simulink model "Integrated_Model"  (R2019a)
settings: Solver=FixedStepAuto  StartTime=0.0  StopTime=1000  FixedStep=0.1  RelTol=1e-3
settings Model: Creator=Kore  LastModifiedBy=User

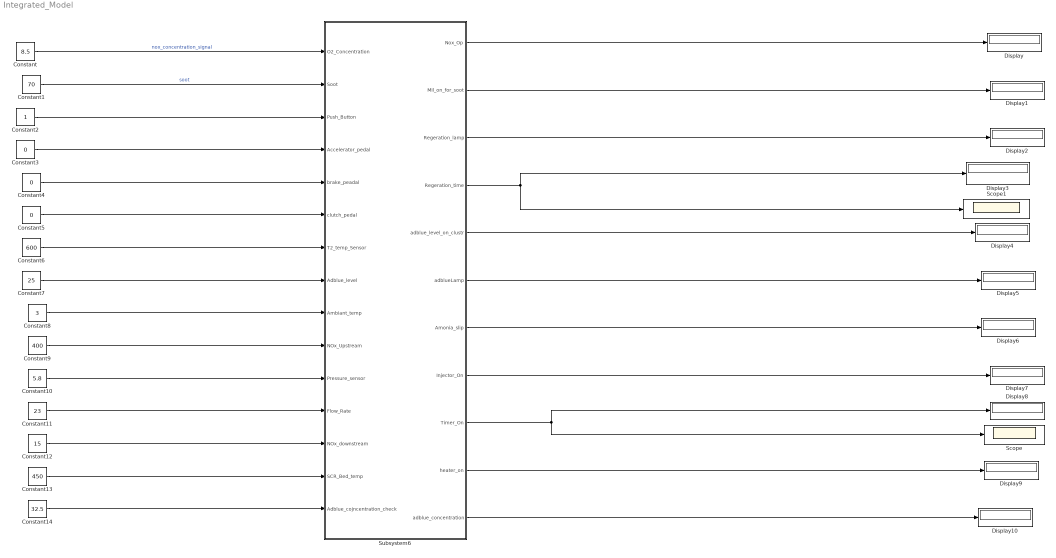
== system Integrated_Model ==
  Constant : Constant  Value=8.5
  Constant1 : Constant  Value=70
  Constant10 : Constant  Value=5.8
  Constant11 : Constant  Value=23
  Constant12 : Constant  Value=15
  Constant13 : Constant  Value=450
  Constant14 : Constant  Value=32.5
  Constant2 : Constant
  Constant3 : Constant  Value=0
  Constant4 : Constant  Value=0
  Constant5 : Constant  Value=0
  Constant6 : Constant  Value=600
  Constant7 : Constant  Value=25
  Constant8 : Constant  Value=3
  Constant9 : Constant  Value=400
  Display{,1..10} (11 alike) : Display
  Scope : Scope
  Scope1 : Scope
  Subsystem6 : Subsystem
  wires:
  Constant/1 -> Subsystem6/1(O2_Concentration)  "nox_concentration_signal"
  Constant1/1 -> Subsystem6/2(Soot)  "soot"
  Constant2/1 -> Subsystem6/3(Push_Button)
  Constant3/1 -> Subsystem6/4(Accelerator_pedal)
  Constant4/1 -> Subsystem6/5(brake_peadal)
  Constant5/1 -> Subsystem6/6(clutch_pedal)
  Constant6/1 -> Subsystem6/7(T2_temp_Sensor)
  Constant7/1 -> Subsystem6/8(Adblue_level)
  Constant8/1 -> Subsystem6/9(Ambiant_temp)
  Constant9/1 -> Subsystem6/10(NOx_Upstream)
  Constant10/1 -> Subsystem6/11(Pressure_sensor)
  Constant11/1 -> Subsystem6/12(Flow_Rate)
  Constant12/1 -> Subsystem6/13(NOx_downstream)
  Constant13/1 -> Subsystem6/14(SCR_Bed_temp)
  Subsystem6/1(Nox_Op) -> Display/1
  Subsystem6/2(MIl_on_for_soot) -> Display1/1
  Subsystem6/3(Regeration_lamp) -> Display2/1
  Subsystem6/4(Regeration_time) -> Scope1/1, Display3/1
  Subsystem6/5(adblue_level_on_clustr) -> Display4/1
  Subsystem6/7(Amonia_slip) -> Display6/1
  Subsystem6/8(Injector_On) -> Display7/1
  Subsystem6/9(Timer_On) -> Display8/1, Scope/1
  Subsystem6/10(heater_on) -> Display9/1
  Subsystem6/11(adblue_concentration) -> Display10/1
  Constant14/1 -> Subsystem6/15(Adblue_cojncentration_check)
  Subsystem6/6(adblueLamp) -> Display5/1

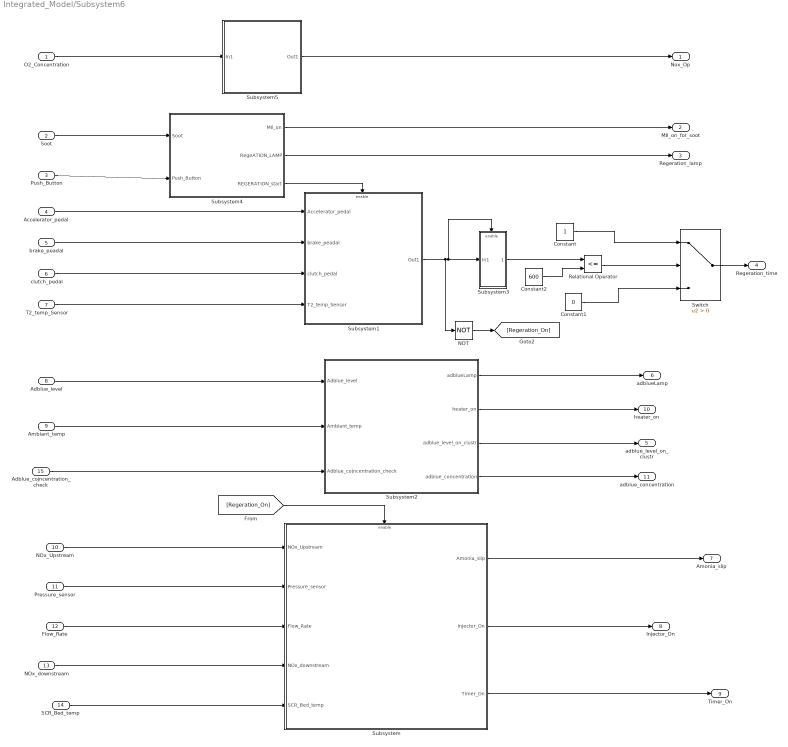
== system Integrated_Model/Subsystem6 ==
  O2_Concentration : Inport
  Soot : Inport  Port=2
  Push_Button : Inport  Port=3
  Accelerator_pedal : Inport  Port=4
  brake_peadal : Inport  Port=5
  clutch_pedal : Inport  Port=6
  T2_temp_Sensor : Inport  Port=7
  Adblue_level : Inport  Port=8
  Ambiant_temp : Inport  Port=9
  NOx_Upstream : Inport  Port=10
  Pressure_sensor : Inport  Port=11
  Flow_Rate : Inport  Port=12
  NOx_downstream : Inport  Port=13
  SCR_Bed_temp : Inport  Port=14
  Adblue_cojncentration_check : Inport  Port=15
  Constant : Constant
  Constant1 : Constant  Value=0
  Constant2 : Constant  Value=600
  NOT : Logic  Operator=NOT  IconShape=distinctive  AllPortsSameDT=off  OutDataTypeStr=boolean
  Relational Operator : RelationalOperator  Operator=<=  OutDataTypeStr=boolean  RndMeth=Simplest
  Subsystem : Subsystem
  Subsystem1 : Subsystem
  Subsystem2 : Subsystem
  Subsystem3 : Subsystem
  Subsystem4 : Subsystem
  Subsystem5 : Subsystem
  Switch : Switch  Criteria=u2 > Threshold
  Nox_Op : Outport
  MIl_on_for_soot : Outport  Port=2
  Regeration_lamp : Outport  Port=3
  Regeration_time : Outport  Port=4
  adblue_level_on_clustr : Outport  Port=5
  adblueLamp : Outport  Port=6
  Amonia_slip : Outport  Port=7
  Injector_On : Outport  Port=8
  Timer_On : Outport  Port=9
  heater_on : Outport  Port=10
  adblue_concentration : Outport  Port=11
  wires:
  T2_temp_Sensor/1 -> Subsystem1/4(T2_temp_Sensor)
  NOT/1 -> [Regeration_On]
  Subsystem/3(Timer_On) -> Timer_On/1
  Subsystem1/1(Out1) -> Subsystem3/Enable, Subsystem3/1(In1), NOT/1
  Push_Button/1 -> Subsystem4/2(Push_Button)
  Subsystem4/3(REGERATION_start) -> Subsystem1/Enable
  Switch/1 -> Regeration_time/1
  Subsystem/1(Amonia_slip) -> Amonia_slip/1
  NOx_Upstream/1 -> Subsystem/1(NOx_Upstream)
  Subsystem3/1(Out1) -> Relational Operator/1
  Subsystem5/1(Out1) -> Nox_Op/1
  Subsystem4/2(RegeATION_LAMP) -> Regeration_lamp/1
  [Regeration_On] -> Subsystem/Enable
  Adblue_level/1 -> Subsystem2/1(Adblue_level)
  O2_Concentration/1 -> Subsystem5/1(In1)
  clutch_pedal/1 -> Subsystem1/3(clutch_pedal)
  Accelerator_pedal/1 -> Subsystem1/1(Accelerator_pedal)
  Flow_Rate/1 -> Subsystem/3(Flow_Rate)
  Soot/1 -> Subsystem4/1(Soot)
  Pressure_sensor/1 -> Subsystem/2(Pressure_sensor)
  Subsystem/2(Injector_On) -> Injector_On/1
  NOx_downstream/1 -> Subsystem/4(NOx_downstream)
  SCR_Bed_temp/1 -> Subsystem/5(SCR_Bed_temp)
  Subsystem4/1(MIl_on) -> MIl_on_for_soot/1
  brake_peadal/1 -> Subsystem1/2("brake_peadal ")
  Ambiant_temp/1 -> Subsystem2/2(Ambiant_temp)
  Subsystem2/1(adblueLamp) -> adblueLamp/1
  Subsystem2/3(adblue_level_on_clustr) -> adblue_level_on_clustr/1
  Subsystem2/2(heater_on) -> heater_on/1
  Relational Operator/1 -> Switch/2
  Constant/1 -> Switch/1
  Constant1/1 -> Switch/3
  Constant2/1 -> Relational Operator/2
  Adblue_cojncentration_check/1 -> Subsystem2/3(Adblue_cojncentration_check)
  Subsystem2/4(adblue_concentration) -> adblue_concentration/1

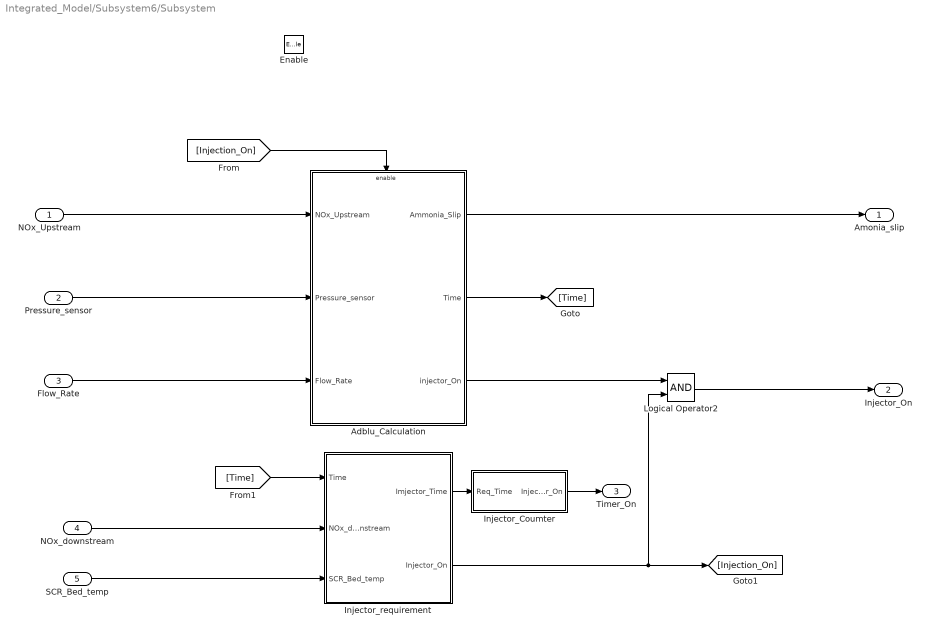
== system Integrated_Model/Subsystem6/Subsystem ==
  NOx_Upstream : Inport
  Pressure_sensor : Inport  Port=2
  Flow_Rate : Inport  Port=3
  NOx_downstream : Inport  Port=4
  SCR_Bed_temp : Inport  Port=5
  Enable : EnablePort
  Adblu_Calculation : Subsystem
  Injector_Coumter : Subsystem
  Injector_requirement : Subsystem
  Logical Operator2 : Logic  AllPortsSameDT=off  OutDataTypeStr=boolean
  Amonia_slip : Outport
  Injector_On : Outport  Port=2
  Timer_On : Outport  Port=3
  wires:
  Adblu_Calculation/2(Time) -> [Time]
  [Time] -> Injector_requirement/1(Time)
  Injector_Coumter/1(Injector_On) -> Timer_On/1
  Logical Operator2/1 -> Injector_On/1
  Injector_requirement/2(Injector_On) -> Logical Operator2/2, [Injection_On]
  Injector_requirement/1(Imjector_Time) -> Injector_Coumter/1(Req_Time)
  Adblu_Calculation/3(injector_On) -> Logical Operator2/1
  [Injection_On] -> Adblu_Calculation/Enable
  Adblu_Calculation/1(Ammonia_Slip) -> Amonia_slip/1
  NOx_downstream/1 -> Injector_requirement/2(NOx_downstream)
  NOx_Upstream/1 -> Adblu_Calculation/1(NOx_Upstream)
  SCR_Bed_temp/1 -> Injector_requirement/3(SCR_Bed_temp)
  Pressure_sensor/1 -> Adblu_Calculation/2(Pressure_sensor)
  Flow_Rate/1 -> Adblu_Calculation/3(Flow_Rate)

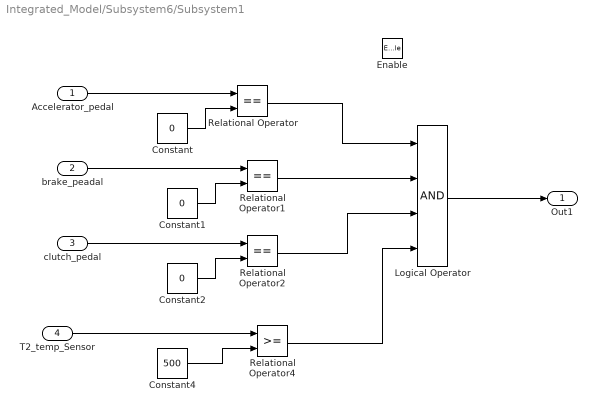
== system Integrated_Model/Subsystem6/Subsystem1 ==
  Accelerator_pedal : Inport
  "brake_peadal " : Inport  Port=2
  clutch_pedal : Inport  Port=3
  T2_temp_Sensor : Inport  Port=4
  Enable : EnablePort  StatesWhenEnabling=reset
  Constant : Constant  Value=0
  Constant1 : Constant  Value=0
  Constant2 : Constant  Value=0
  Constant4 : Constant  Value=500
  Logical Operator : Logic  Inputs=4  AllPortsSameDT=off  OutDataTypeStr=boolean
  Relational Operator : RelationalOperator  Operator===  OutDataTypeStr=boolean  RndMeth=Simplest
  Relational Operator1 : RelationalOperator  Operator===  OutDataTypeStr=boolean  RndMeth=Simplest
  Relational Operator2 : RelationalOperator  Operator===  OutDataTypeStr=boolean  RndMeth=Simplest
  Relational Operator4 : RelationalOperator  OutDataTypeStr=boolean  RndMeth=Simplest
  Out1 : Outport
  wires:
  Constant/1 -> Relational Operator/2
  Accelerator_pedal/1 -> Relational Operator/1
  "brake_peadal "/1 -> Relational Operator1/1
  Constant1/1 -> Relational Operator1/2
  Constant2/1 -> Relational Operator2/2
  clutch_pedal/1 -> Relational Operator2/1
  Relational Operator/1 -> Logical Operator/1
  Relational Operator1/1 -> Logical Operator/2
  Relational Operator2/1 -> Logical Operator/3
  T2_temp_Sensor/1 -> Relational Operator4/1
  Constant4/1 -> Relational Operator4/2
  Logical Operator/1 -> Out1/1
  Relational Operator4/1 -> Logical Operator/4

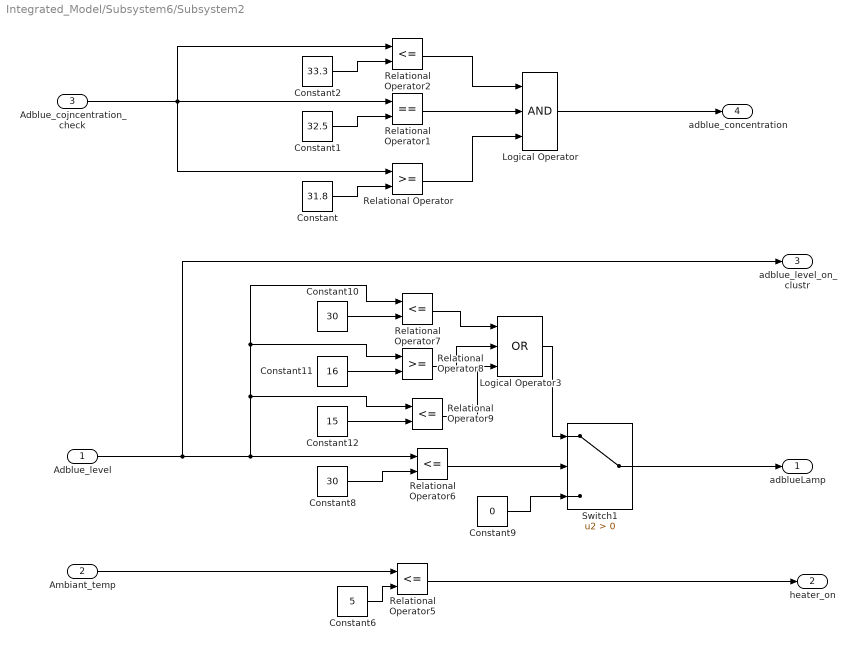
== system Integrated_Model/Subsystem6/Subsystem2 ==
  Adblue_level : Inport
  Ambiant_temp : Inport  Port=2
  Adblue_cojncentration_check : Inport  Port=3
  Constant : Constant  Value=31.8
  Constant1 : Constant  Value=32.5
  Constant10 : Constant  Value=30
  Constant11 : Constant  Value=16
  Constant12 : Constant  Value=15
  Constant2 : Constant  Value=33.3
  Constant6 : Constant  Value=5  OutDataTypeStr=int8
  Constant8 : Constant  Value=30
  Constant9 : Constant  Value=0
  Logical Operator : Logic  Inputs=3  AllPortsSameDT=off  OutDataTypeStr=boolean
  Logical Operator3 : Logic  Operator=OR  Inputs=3  AllPortsSameDT=off  OutDataTypeStr=boolean
  Relational Operator : RelationalOperator  OutDataTypeStr=boolean  RndMeth=Simplest
  Relational Operator1 : RelationalOperator  Operator===  OutDataTypeStr=boolean  RndMeth=Simplest
  Relational Operator{2,5..7,9} (5 alike) : RelationalOperator  Operator=<=  OutDataTypeStr=boolean  RndMeth=Simplest
  Relational Operator8 : RelationalOperator  OutDataTypeStr=boolean  RndMeth=Simplest
  Switch1 : Switch  Criteria=u2 > Threshold
  adblueLamp : Outport
  heater_on : Outport  Port=2
  adblue_level_on_clustr : Outport  Port=3
  adblue_concentration : Outport  Port=4
  wires:
  Logical Operator3/1 -> Switch1/1
  Constant9/1 -> Switch1/3
  Adblue_level/1 -> adblue_level_on_clustr/1, Relational Operator6/1, Relational Operator9/1, Relational Operator8/1, Relational Operator7/1
  Constant10/1 -> Relational Operator7/2
  Constant11/1 -> Relational Operator8/2
  Constant8/1 -> Relational Operator6/2
  Relational Operator8/1 -> Logical Operator3/2
  Constant12/1 -> Relational Operator9/2
  Relational Operator9/1 -> Logical Operator3/3
  Relational Operator6/1 -> Switch1/2
  Relational Operator7/1 -> Logical Operator3/1
  Constant6/1 -> Relational Operator5/2
  Relational Operator5/1 -> heater_on/1
  Switch1/1 -> adblueLamp/1
  Ambiant_temp/1 -> Relational Operator5/1
  Constant/1 -> Relational Operator/2
  Constant1/1 -> Relational Operator1/2
  Adblue_cojncentration_check/1 -> Relational Operator/1, Relational Operator2/1, Relational Operator1/1
  Constant2/1 -> Relational Operator2/2
  Relational Operator2/1 -> Logical Operator/1
  Relational Operator1/1 -> Logical Operator/2
  Relational Operator/1 -> Logical Operator/3
  Logical Operator/1 -> adblue_concentration/1

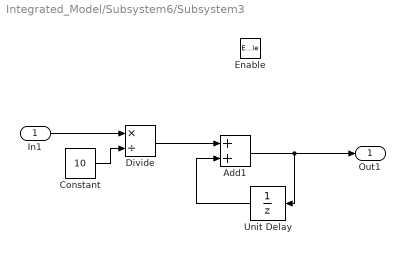
== system Integrated_Model/Subsystem6/Subsystem3 ==
  In1 : Inport
  Enable : EnablePort  StatesWhenEnabling=reset
  Add1 : Sum  OutDataTypeStr=double  RndMeth=Round
  Constant : Constant  Value=10
  Divide : Product  Inputs=*/
  Unit Delay : UnitDelay  InitialCondition=0.1  SampleTime=-1  HasFrameUpgradeWarning=on
  Out1 : Outport
  wires:
  Add1/1 -> Out1/1, Unit Delay/1
  Unit Delay/1 -> Add1/2
  In1/1 -> Divide/1
  Divide/1 -> Add1/1
  Constant/1 -> Divide/2

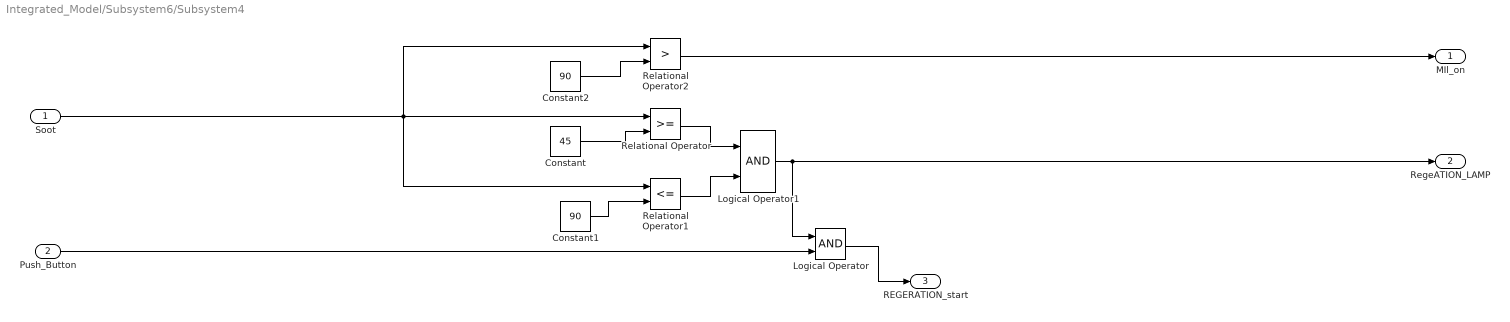
== system Integrated_Model/Subsystem6/Subsystem4 ==
  Soot : Inport
  Push_Button : Inport  Port=2
  Constant : Constant  Value=45
  Constant1 : Constant  Value=90
  Constant2 : Constant  Value=90
  Logical Operator : Logic  AllPortsSameDT=off  OutDataTypeStr=boolean
  Logical Operator1 : Logic  AllPortsSameDT=off  OutDataTypeStr=boolean
  Relational Operator : RelationalOperator  OutDataTypeStr=boolean  RndMeth=Simplest
  Relational Operator1 : RelationalOperator  Operator=<=  OutDataTypeStr=boolean  RndMeth=Simplest
  Relational Operator2 : RelationalOperator  Operator=>  OutDataTypeStr=boolean  RndMeth=Simplest
  MIl_on : Outport
  RegeATION_LAMP : Outport  Port=2
  REGERATION_start : Outport  Port=3
  wires:
  Soot/1 -> Relational Operator1/1, Relational Operator2/1, Relational Operator/1
  Logical Operator/1 -> REGERATION_start/1
  Logical Operator1/1 -> RegeATION_LAMP/1, Logical Operator/1
  Constant2/1 -> Relational Operator2/2
  Push_Button/1 -> Logical Operator/2
  Constant1/1 -> Relational Operator1/2
  Constant/1 -> Relational Operator/2
  Relational Operator1/1 -> Logical Operator1/2
  Relational Operator2/1 -> MIl_on/1
  Relational Operator/1 -> Logical Operator1/1

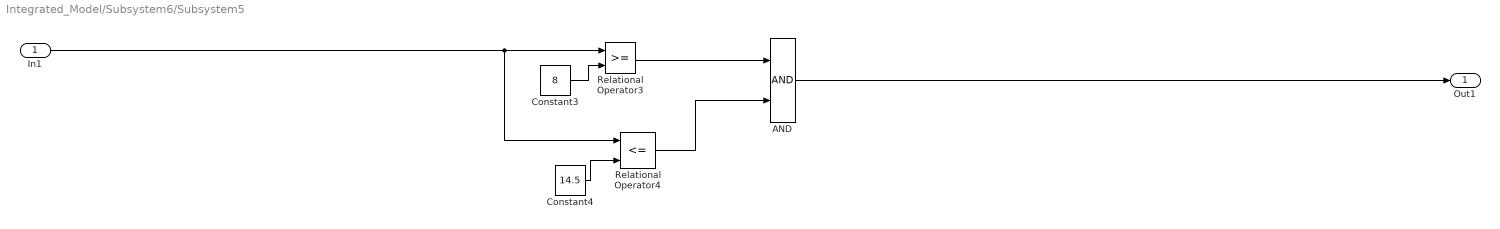
== system Integrated_Model/Subsystem6/Subsystem5 ==
  In1 : Inport
  AND : Logic  AllPortsSameDT=off  OutDataTypeStr=boolean
  Constant3 : Constant  Value=8
  Constant4 : Constant  Value=14.5
  Relational Operator3 : RelationalOperator  OutDataTypeStr=boolean  RndMeth=Simplest
  Relational Operator4 : RelationalOperator  Operator=<=  OutDataTypeStr=boolean  RndMeth=Simplest
  Out1 : Outport
  wires:
  Constant3/1 -> Relational Operator3/2
  Relational Operator3/1 -> AND/1
  AND/1 -> Out1/1
  In1/1 -> Relational Operator4/1, Relational Operator3/1
  Constant4/1 -> Relational Operator4/2
  Relational Operator4/1 -> AND/2

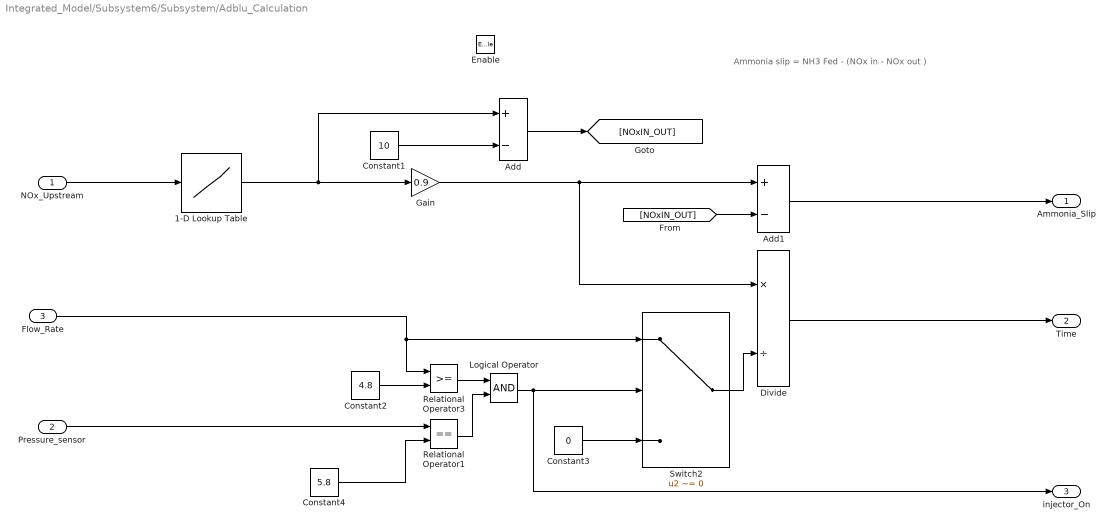
== system Integrated_Model/Subsystem6/Subsystem/Adblu_Calculation ==
  note: Ammonia slip = NH3 Fed - (NOx in - NOx out )
  NOx_Upstream : Inport
  Pressure_sensor : Inport  Port=2
  Flow_Rate : Inport  Port=3
  Enable : EnablePort  StatesWhenEnabling=reset
  1-D Lookup Table : Lookup_n-D  NumberOfTableDimensions=1  BreakpointsForDimension1=|  BreakpointsForDimension1DataTypeStr=double  Table=|  TableDataTypeStr=double  IntermediateResultsDataTypeStr=double  InternalRulePriority=Speed  OutDataTypeStr=double  RndMeth=Simplest  FractionDataTypeStr=double  InputSameDT=on
      BreakpointsForDimension1=|
      | [10
      | 70
      | 77.6
      | 80.4
      | 86.4
      | 99.6
      | 108
      | 117.6
      | 127.2
      | 136.8
      | 149.3
      | 158.3
      | 163.3
      | 168.3
      | 175.3
      | 181.5
      | 187.7
      | 193.9
      | 200.1
      | 206.3
      | 212.85
      | 223.5
      | 233.15
      | 242.8
      | 255.45
      | 264.9
      | 275.35
      | 285.8
      | 296.25
      | 306.7
      | 317.15
      | 327.6
      | 338.05
      | 348.5
      | 358.95
      | 369.4
      | 379.85
      | 390.3
      | 400.75
      | 411.2
      | 421.65
      | 432.1
      | 442.55
      | 453
      | 463.45
      | 473.9
      | 484.35
      | 494.8
      | 505.25
      | 515.7
      | 526.15
      | 536.6
      | 547.05
      | 557.5
      | 567.95
      | 578.4
      | 588.85
      | 599.3
      | 609.75
      | 620.2
      | 630.65
      | 641.1
      | 651.55
      | 662
      | 672.45
      | 682.9
      | 693.35
      | 703.8
      | ]
      Table=|
      | [10
      | 70
      | 77.6
      | 80.4
      | 86.4
      | 99.6
      | 108
      | 117.6
      | 127.2
      | 136.8
      | 149.3
      | 158.3
      | 163.3
      | 168.3
      | 175.3
      | 181.5
      | 187.7
      | 193.9
      | 200.1
      | 206.3
      | 212.85
      | 223.5
      | 233.15
      | 242.8
      | 255.45
      | 264.9
      | 275.35
      | 285.8
      | 296.25
      | 306.7
      | 317.15
      | 327.6
      | 338.05
      | 348.5
      | 358.95
      | 369.4
      | 379.85
      | 390.3
      | 400.75
      | 411.2
      | 421.65
      | 432.1
      | 442.55
      | 453
      | 463.45
      | 473.9
      | 484.35
      | 494.8
      | 505.25
      | 515.7
      | 526.15
      | 536.6
      | 547.05
      | 557.5
      | 567.95
      | 578.4
      | 588.85
      | 599.3
      | 609.75
      | 620.2
      | 630.65
      | 641.1
      | 651.55
      | 662
      | 672.45
      | 682.9
      | 693.35
      | 703.8
      | ]
  Add : Sum  Inputs=+-
  Add1 : Sum  Inputs=+-
  Constant1 : Constant  Value=10
  Constant2 : Constant  Value=4.8
  Constant3 : Constant  Value=0
  Constant4 : Constant  Value=5.8
  Divide : Product  Inputs=*/  OutDataTypeStr=double  RndMeth=Round
  Gain : Gain  Gain=0.9
  Logical Operator : Logic  AllPortsSameDT=off  OutDataTypeStr=boolean
  Relational Operator1 : RelationalOperator  Operator===  OutDataTypeStr=boolean  RndMeth=Simplest
  Relational Operator3 : RelationalOperator  OutDataTypeStr=boolean  RndMeth=Simplest
  Switch2 : Switch  Criteria=u2 ~= 0
  Ammonia_Slip : Outport
  Time : Outport  Port=2
  injector_On : Outport  Port=3
  wires:
  Pressure_sensor/1 -> Relational Operator1/1
  Add/1 -> [NOxIN_OUT]
  Constant1/1 -> Add/2
  Relational Operator1/1 -> Logical Operator/2
  Constant4/1 -> Relational Operator1/2
  NOx_Upstream/1 -> 1-D Lookup Table/1
  Constant2/1 -> Relational Operator3/2
  Relational Operator3/1 -> Logical Operator/1
  Constant3/1 -> Switch2/3
  Switch2/1 -> Divide/2
  Logical Operator/1 -> injector_On/1, Switch2/2
  [NOxIN_OUT] -> Add1/2
  Flow_Rate/1 -> Relational Operator3/1, Switch2/1
  Add1/1 -> Ammonia_Slip/1
  Gain/1 -> Divide/1, Add1/1
  Divide/1 -> Time/1
  1-D Lookup Table/1 -> Gain/1, Add/1

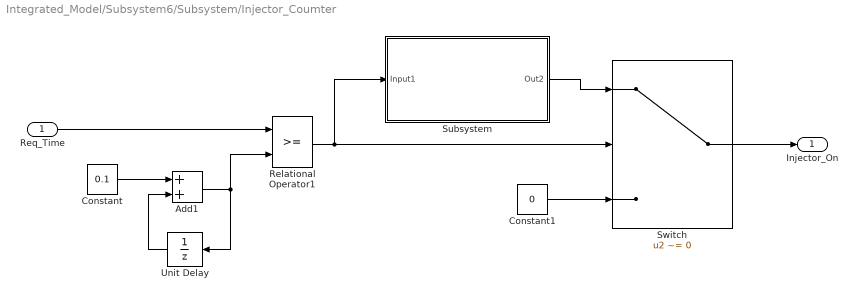
== system Integrated_Model/Subsystem6/Subsystem/Injector_Coumter ==
  Req_Time : Inport
  Add1 : Sum
  Constant : Constant  Value=0.1
  Constant1 : Constant  Value=0
  Relational Operator1 : RelationalOperator  OutDataTypeStr=boolean  RndMeth=Simplest
  Subsystem : Subsystem
  Switch : Switch  Criteria=u2 ~= 0
  Unit Delay : UnitDelay  SampleTime=-1  HasFrameUpgradeWarning=on
  Injector_On : Outport
  wires:
  Constant1/1 -> Switch/3
  Unit Delay/1 -> Add1/2
  Constant/1 -> Add1/1
  Add1/1 -> Unit Delay/1, Relational Operator1/2
  Subsystem/1(Out2) -> Switch/1
  Req_Time/1 -> Relational Operator1/1
  Switch/1 -> Injector_On/1
  Relational Operator1/1 -> Subsystem/1(Input1), Switch/2

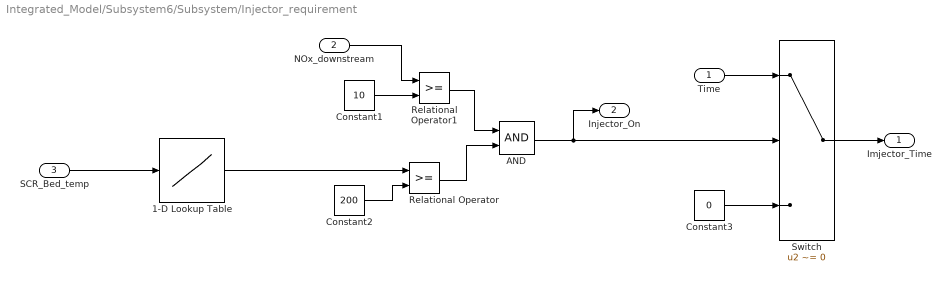
== system Integrated_Model/Subsystem6/Subsystem/Injector_requirement ==
  Time : Inport
  NOx_downstream : Inport  Port=2
  SCR_Bed_temp : Inport  Port=3
  1-D Lookup Table : Lookup_n-D  NumberOfTableDimensions=1  BreakpointsForDimension1=[1:10:650]  BreakpointsForDimension2=[1:1:500]  BreakpointsForDimension1DataTypeStr=double  Table=[1:10:650]  TableDataTypeStr=double  IntermediateResultsDataTypeStr=double  InternalRulePriority=Speed  OutDataTypeStr=double  RndMeth=Simplest  FractionDataTypeStr=double  InputSameDT=on
  AND : Logic  AllPortsSameDT=off  OutDataTypeStr=boolean
  Constant1 : Constant  Value=10
  Constant2 : Constant  Value=200
  Constant3 : Constant  Value=0
  Relational Operator : RelationalOperator  OutDataTypeStr=boolean  RndMeth=Simplest
  Relational Operator1 : RelationalOperator  OutDataTypeStr=boolean  RndMeth=Simplest
  Switch : Switch  Criteria=u2 ~= 0
  Imjector_Time : Outport
  Injector_On : Outport  Port=2
  wires:
  Constant1/1 -> Relational Operator1/2
  Constant2/1 -> Relational Operator/2
  Constant3/1 -> Switch/3
  1-D Lookup Table/1 -> Relational Operator/1
  AND/1 -> Injector_On/1, Switch/2
  Time/1 -> Switch/1
  Relational Operator1/1 -> AND/1
  Relational Operator/1 -> AND/2
  SCR_Bed_temp/1 -> 1-D Lookup Table/1
  Switch/1 -> Imjector_Time/1
  NOx_downstream/1 -> Relational Operator1/1

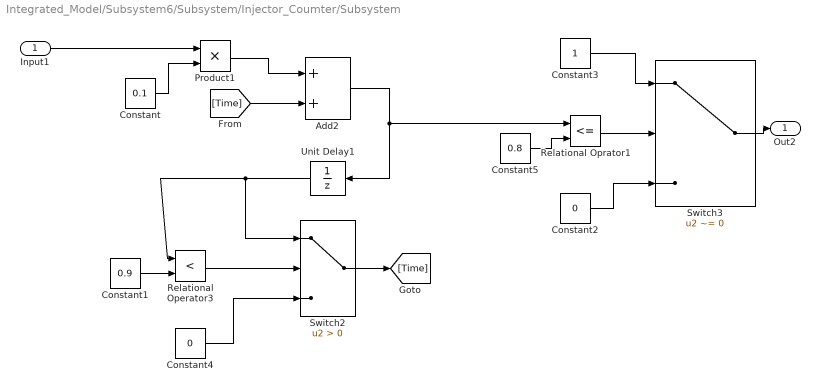
== system Integrated_Model/Subsystem6/Subsystem/Injector_Coumter/Subsystem ==
  Input1 : Inport
  Add2 : Sum
  Constant : Constant  Value=0.1
  Constant1 : Constant  Value=0.9
  Constant2 : Constant  Value=0
  Constant3 : Constant
  Constant4 : Constant  Value=0
  Constant5 : Constant  Value=0.8
  Product1 : Product
  Relational Operator3 : RelationalOperator  Operator=<  OutDataTypeStr=boolean  RndMeth=Simplest
  Relational Oprator1 : RelationalOperator  Operator=<=  OutDataTypeStr=boolean  RndMeth=Simplest
  Switch2 : Switch  Criteria=u2 > Threshold
  Switch3 : Switch  Criteria=u2 ~= 0
  Unit Delay1 : UnitDelay  SampleTime=-1  HasFrameUpgradeWarning=on
  Out2 : Outport
  wires:
  Unit Delay1/1 -> Relational Operator3/1, Switch2/1
  Relational Operator3/1 -> Switch2/2
  Constant3/1 -> Switch3/1
  Switch3/1 -> Out2/1
  Constant5/1 -> Relational Oprator1/2
  Constant/1 -> Product1/2
  Switch2/1 -> [Time]
  Product1/1 -> Add2/1
  Constant1/1 -> Relational Operator3/2
  Constant4/1 -> Switch2/3
  Input1/1 -> Product1/1
  Constant2/1 -> Switch3/3
  [Time] -> Add2/2
  Relational Oprator1/1 -> Switch3/2
  Add2/1 -> Relational Oprator1/1, Unit Delay1/1
